simulink model "step6_2_controller_feedback_test1"  (R2021b)
settings: Solver=VariableStepAuto  StartTime=0.0  StopTime=10.0  RelTol=1e-3
values from neighbouring files (symbols this model uses):
  A = [0 1 0 0 ... (first row only)    [linearize_script.m]    (also in step4_0_linearize_operating_point.m = double(A); step4_linearized_system.mat = [0 0.182757622438 0 -107.203412441 0 1 -70.6718613709 0 147.; syms_test.m = double(A))
  B = [0 ... (first row only)    [linearize_script.m]    (also in step4_0_linearize_operating_point.m = double(B); step4_linearized_system.mat = [0 0 0 0 2608.67338972]; syms_test.m = double(B))
  C = [1 0 0 0 ... (first row only)    [linearize_script.m]    (also in matrixmaker_linearization.m = [b_1_0 - P_3 * theta_d_2 * sin(theta_2)  -P_3 * (theta_d_1 +; step4_0_linearize_operating_point.m = [1 0 0 0 0; step4_linearized_system.mat = [1  0  0  0  0; 0  0  1  0  0]; syms_test.m)
  D = zeros(2,1)    [linearize_script.m]    (also in step4_0_linearize_operating_point.m; step4_linearized_system.mat = [0 0]; syms_test.m)
  g1 = (m_1 * c_1_0 + m_2 * l_1) * g    [compare_ourmodel_with_others.m]    (also in step2_whitebox_beam.m; step4_0_linearize_operating_point.m = (m1 * c1 + m2 * l1) * g; step5_observor_design.m = (m1 * c1 + m2 * l1) * g; step6_1_controller_feedback.m = (m1 * c1 + m2 * l1) * g)
  g2 = m_2 * c_2_0 * g    [compare_ourmodel_with_others.m]    (also in step2_whitebox_beam.m; step4_0_linearize_operating_point.m = m2 * c2 * g; step5_observor_design.m = m2 * c2 * g; step6_1_controller_feedback.m = m2 * c2 * g)
  K = K1    [step6_1_controller_feedback.m]
  Ke = [354.974544838  -25.0111429308; 25988.2816466  -5367.91612622; 16.163382401  409.154611883; 13828.3876591  42696.3634009; 71318.1002949  -26510.3632323]    [step5_observor.mat]    (also in step5_observor_design.m = place(A_, B_, 0.5*J)')
  P1 = m_1 * c_1_0 * c_1_0 + m_2 * l_1 * l_1 + I_1_0    [compare_ourmodel_with_others.m]    (also in script_for_test.m = P2(1:L/2+1); step2_whitebox_beam.m; step4_0_linearize_operating_point.m = m1 * c1 * c1 + m2 * l1 * l1 + I1; step5_observor_design.m = m1 * c1 * c1 + m2 * l1 * l1 + I1)
  P2 = m_2 * c_2_0 * c_2_0 + I_2_0    [compare_ourmodel_with_others.m]    (also in script_for_test.m = abs(Y/L); step2_whitebox_beam.m; step4_0_linearize_operating_point.m = m2 * c2 * c2 + I2; step5_observor_design.m = m2 * c2 * c2 + I2)
  P3 = m_2 * l_1 * c_2_0    [compare_ourmodel_with_others.m]    (also in step2_whitebox_beam.m; step4_0_linearize_operating_point.m = m2 * l1 * c2; step5_observor_design.m = m2 * l1 * c2; step6_1_controller_feedback.m = m2 * l1 * c2)
  params = [-0.0300000121036330, 0.0303451968350115, 0.1000000000017210, 1.00882387117299e-05, 10.27570530021582, 1.78577414601457e-05, 65.9998023466922, 0.01300000000002200]    [compare_ourmodel_with_others.m]    (also in linearization.m = params_hat; matrixmaker_linearization.m = [-0.001, 0.077, 0.2, 0.00004, 20.684, 0.0004, 15, 0.03]; params.mat = [9.81 0.1 0.1 0.125 0.046955 -0.032 0.04609 0.0888 9.9e-05 6; sss.m = [9.81, 0.1, 0.1, 0.125, 0.04824, -0.041443, .0607558, 0.1154)
  theta_1_0 = pi    (= 3.14159265359)    [hwinit.m]    (also in hwinit_raw.m; step4_0_linearize_operating_point.m; step5_observor_design.m = x_op(1); step6_1_controller_feedback.m = x_op(1))
  theta_2_0 = 0    [hwinit.m]    (also in hwinit_raw.m; step4_0_linearize_operating_point.m; step5_observor_design.m = x_op(3); step6_1_controller_feedback.m = x_op(3))
  x_op_relative = [0; 0; 0; 0; 0]    [step5_observor_design.m]    (also in step6_1_controller_feedback.m)
settings Model: LastModifiedBy=lyitingli
settings OptimizationCC: BlockReduction=off  BooleanDataType=off
settings DebuggingCC: SaveWithParameterizedLinksMsg=none  UnderspecifiedInitializationDetection=Classic  MergeDetectMultiDrivingBlocksExec=none  SignalResolutionControl=TryResolveAllWithWarning
settings HardwareCC: TargetUnknown=on
settings ModelReferenceCC: PropagateSignalLabelsOutOfModel=off

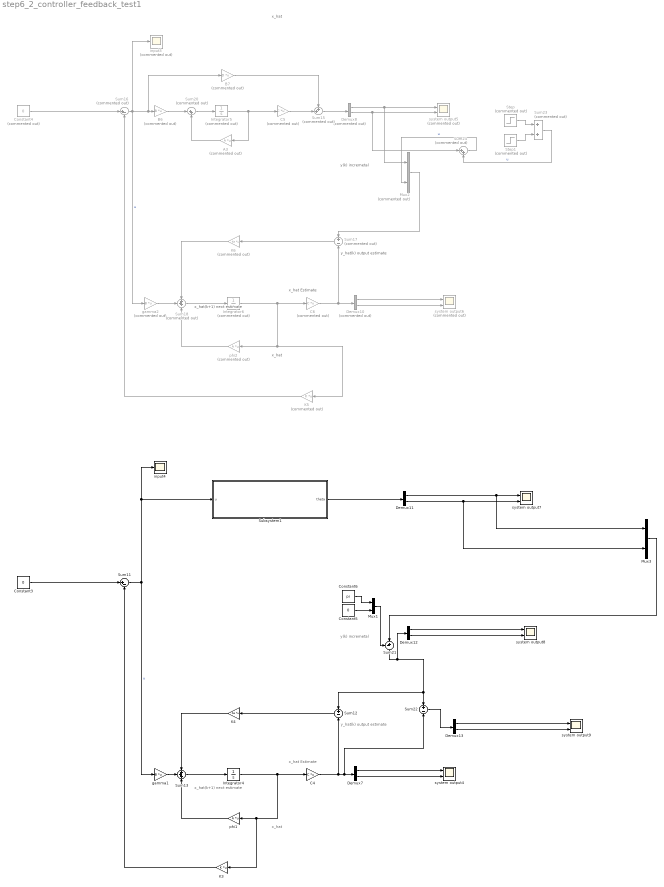
== system step6_2_controller_feedback_test1 ==
  note: x_hat
  note: y_hat(k)
      | output estimate
  note: x_hat
  note: y(k)
      | incremetal
  note: x_hat(k+1)
      | next estimate
  note: x_hat
      | Estimate
  note: y_hat(k)
      | output estimate
  note: x_hat
  note: y(k)
      | incremetal
  note: x_hat(k+1)
      | next estimate
  note: x_hat
      | Estimate
  A3 : Gain  Commented=on  Gain=A  Multiplication=Matrix(K*u) (u vector)
  B6 : Gain  Commented=on  Gain=B  Multiplication=Matrix(K*u)
  B7 : Gain  Commented=on  Gain=D  Multiplication=Matrix(K*u)
  C4 : Gain  Gain=C  Multiplication=Matrix(K*u) (u vector)
  C5 : Gain  Commented=on  Gain=C  Multiplication=Matrix(K*u) (u vector)
  C6 : Gain  Commented=on  Gain=C  Multiplication=Matrix(K*u) (u vector)
  Constant3 : Constant  Value=0  SampleTime=0.001
  Constant4 : Constant  Commented=on  Value=0  SampleTime=0.001
  Constant5 : Constant  Value=0  SampleTime=-1
  Constant6 : Constant  Value=pi  SampleTime=-1
  Demux10 : Demux  Commented=on  Outputs=2
  Demux{7,11..13} (4 alike) : Demux  Outputs=2
  Demux8 : Demux  Commented=on  Outputs=2
  Integrator4 : Integrator  InitialCondition=x_op_relative
  Integrator5 : Integrator  Commented=on  InitialCondition=x_op_relative
  Integrator6 : Integrator  Commented=on  InitialCondition=x_op_relative
  K3 : Gain  Gain=K  Multiplication=Matrix(K*u) (u vector)
  K4 : Gain  Gain=Ke  Multiplication=Matrix(K*u) (u vector)
  K5 : Gain  Commented=on  Gain=K  Multiplication=Matrix(K*u) (u vector)
  K6 : Gain  Commented=on  Gain=Ke  Multiplication=Matrix(K*u) (u vector)
  Mux1 : Mux  Inputs=2
  Mux2 : Mux  Commented=on  Inputs=2
  Mux3 : Mux  Inputs=2
  Step : Step  Commented=on  After=0  SampleTime=0
  Step1 : Step  Commented=on  Time=1.05  After=0  SampleTime=0
  Subsystem1 : Subsystem
  Sum11 : Sum  Inputs=|+-
  Sum12 : Sum  Inputs=+|-
  Sum13 : Sum  Inputs=+++
  Sum15 : Sum  Commented=on  Inputs=++|
  Sum16 : Sum  Commented=on  Inputs=|+-
  Sum17 : Sum  Commented=on  Inputs=+|-
  Sum18 : Sum  Commented=on  Inputs=+++
  Sum20 : Sum  Commented=on  Inputs=|++
  Sum21 : Sum  Inputs=-+|
  Sum22 : Sum  Inputs=+|-
  Sum23 : Sum  Commented=on
  Sum24 : Sum  Commented=on  Inputs=|++
  gamma1 : Gain  Gain=B  Multiplication=Matrix(K*u)
  gamma2 : Gain  Commented=on  Gain=B  Multiplication=Matrix(K*u)
  input3 : Scope  Commented=on
  input4 : Scope
  phi1 : Gain  Gain=A  Multiplication=Matrix(K*u) (u vector)
  phi2 : Gain  Commented=on  Gain=A  Multiplication=Matrix(K*u) (u vector)
  system output{4,7..9} (4 alike) : Scope  NumInputPorts=2
  system output5 : Scope  Commented=on  NumInputPorts=2
  system output6 : Scope  Commented=on  NumInputPorts=2
  wires:
  Demux7/1 -> system output4/1
  Demux7/2 -> system output4/2
  C4/1 -> Sum12/2, Sum22/2, Demux7/1
  phi1/1 -> Sum13/3
  Sum12/1 -> K4/1
  Sum13/1 -> Integrator4/1
  K4/1 -> Sum13/1
  gamma1/1 -> Sum13/2
  Integrator4/1 -> phi1/1, K3/1, C4/1
  Sum11/1 -> Subsystem1/1(u), input4/1, gamma1/1  "u"
  Constant3/1 -> Sum11/1
  K3/1 -> Sum11/2
  B7/1 -> Sum15/1
  Integrator5/1 -> A3/1, C5/1
  Demux8/1 -> Mux2/1, system output5/1
  Demux8/2 -> Sum24/1, system output5/2
  K5/1 -> Sum16/2
  C5/1 -> Sum15/2
  Constant4/1 -> Sum16/1
  Sum20/1 -> Integrator5/1
  Sum16/1 -> input3/1, gamma2/1, B7/1, B6/1  "u"
  B6/1 -> Sum20/1
  A3/1 -> Sum20/2
  Integrator6/1 -> C6/1, K5/1, phi2/1
  gamma2/1 -> Sum18/2
  K6/1 -> Sum18/1
  Sum18/1 -> Integrator6/1
  Sum17/1 -> K6/1
  Sum15/1 -> Demux8/1
  phi2/1 -> Sum18/3
  C6/1 -> Demux10/1, Sum17/2
  Demux10/2 -> system output6/2
  Demux10/1 -> system output6/1
  Constant6/1 -> Mux1/1
  Constant5/1 -> Mux1/2
  Mux1/1 -> Sum21/1
  Sum21/1 -> Sum12/1, Sum22/1, Demux12/1
  Demux12/1 -> system output8/1
  Demux12/2 -> system output8/2
  Sum22/1 -> Demux13/1
  Demux13/2 -> system output9/2
  Demux13/1 -> system output9/1
  Mux2/1 -> Sum17/1
  Step/1 -> Sum23/1
  Step1/1 -> Sum23/2
  Sum23/1 -> Sum24/2  "u"
  Sum24/1 -> Mux2/2  "u"
  Demux11/2 -> Mux3/2, system output7/2
  Demux11/1 -> Mux3/1, system output7/1
  Mux3/1 -> Sum21/2
  Subsystem1/1(theta) -> Demux11/1

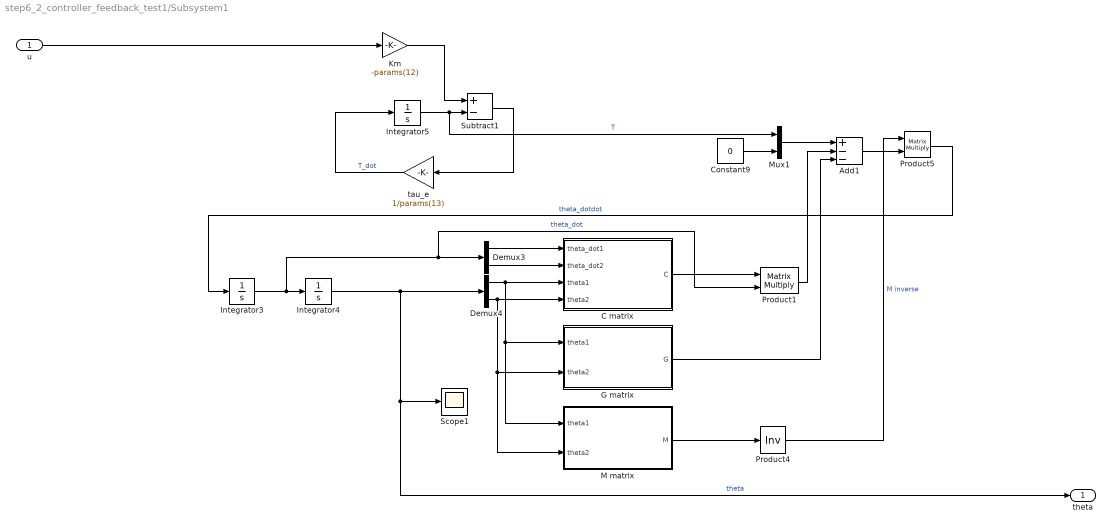
== system step6_2_controller_feedback_test1/Subsystem1 ==
  u : Inport
  Add1 : Sum  Inputs=+--
  C matrix : MATLAB Function  TreatAsAtomicUnit=on
  Constant9 : Constant  Value=0
  Demux3 : Demux  Outputs=2
  Demux4 : Demux  Outputs=2
  G matrix : MATLAB Function  TreatAsAtomicUnit=on
  Integrator3 : Integrator
  Integrator4 : Integrator  InitialCondition=[theta_1_0 theta_2_0]
  Integrator5 : Integrator
  Km : Gain  Gain=-params(12)
  M matrix : MATLAB Function  TreatAsAtomicUnit=on
  Mux1 : Mux  Inputs=2
  Product1 : Product  Inputs=**  Multiplication=Matrix(*)
  Product4 : Product  Inputs=/  Multiplication=Matrix(*)
  Product5 : Product  Inputs=**  Multiplication=Matrix(*)
  Scope1 : Scope
  Subtract1 : Sum  Inputs=+-
  tau_e : Gain  Gain=1/params(13)
  theta : Outport
  wires:
  Demux4/1 -> M matrix/1(theta1), G matrix/1(theta1), C matrix/3(theta1)
  tau_e/1 -> Integrator5/1  "T_dot"
  Constant9/1 -> Mux1/2
  Demux3/1 -> C matrix/1(theta_dot1)
  Add1/1 -> Product5/2
  Subtract1/1 -> tau_e/1
  G matrix/1(G) -> Add1/3
  Integrator3/1 -> Product1/2, Demux3/1, Integrator4/1  "theta_dot"
  C matrix/1(C) -> Product1/1
  Mux1/1 -> Add1/1
  Integrator5/1 -> Mux1/1, Subtract1/2  "T"
  u/1 -> Km/1
  Product5/1 -> Integrator3/1  "theta_dotdot"
  Demux3/2 -> C matrix/2(theta_dot2)
  Integrator4/1 -> Demux4/1, theta/1, Scope1/1  "theta"
  M matrix/1(M) -> Product4/1
  Demux4/2 -> M matrix/2(theta2), G matrix/2(theta2), C matrix/4(theta2)
  Product4/1 -> Product5/1  "M inverse"
  Product1/1 -> Add1/2
  Km/1 -> Subtract1/1

== matlab function step6_2_controller_feedback_test1/Subsystem1/C matrix ==
  data: theta_dot1 input; theta_dot2 input; theta1 input; theta2 input; C output; params parameter; P3 parameter
function C = C(theta_dot1, theta_dot2, theta1, theta2, params, P3)
c00 = params(10) - P3 * theta_dot2 * sin(theta2);
c01 = -P3 * (theta_dot1 + theta_dot2) * sin(theta2);
c10 = P3 * theta_dot1 * sin(theta2);
c11 = params(11);

C = [c00 c01;
     c10 c11];

== matlab function step6_2_controller_feedback_test1/Subsystem1/G matrix ==
  data: theta1 input; theta2 input; G output; g1 parameter; g2 parameter
function G = G(theta1, theta2, g1, g2)
G00 = -g1 * sin(theta1) - g2 * sin(theta1 + theta2);
G01 = -g2 * sin(theta1 + theta2);

G = [G00 G01];

== matlab function step6_2_controller_feedback_test1/Subsystem1/M matrix ==
  data: theta1 input; theta2 input; M output; P1 parameter; P2 parameter; P3 parameter
function M = fcn(theta1, theta2, P1, P2, P3)
M00 = P1 + P2 + 2 * P3 * cos(theta2);
M01 = P2 + P3 * cos(theta2);
M10 = M01;
M11 = P2;

M = [M00 M01;
     M10 M11];
